simulink model "ThermalRct"  (R2023b)
settings: Solver=FixedStepAuto  StartTime=0.0  StopTime=10.0  RelTol=1e-3
settings Model: DataDictionary=ThermalRct.sldd  Creator=84339  LastModifiedBy=84339
settings OptimizationCC: DefaultParameterBehavior=Inlined  EnhancedBackFolding=on  PassReuseOutputArgsAs=Individual arguments  ZeroExternalMemoryAtStartup=off  ZeroInternalMemoryAtStartup=off  OptimizeBlockOrder=speed  DifferentSizesBufferReuse=on  OptimizationCustomize=off  EfficientTunableParamExpr=on
settings DebuggingCC: ParameterTunabilityLossMsg=error
settings ModelReferenceCC: ModelReferenceNumInstancesAllowed=Single
settings SFSimCC: MATLABDynamicMemAlloc=off
settings RTWCC: Description=Embedded Coder  SystemTargetFile=ert.tlc  EmbeddedCoderDictionary=ASW.sldd  GenCodeOnly=on  TemplateMakefile=ert_default_tmf  DataTypeReplacement=CDataTypesFixedWidth
settings CodeAppCC: ForceParamTrailComments=on  IgnoreCustomStorageClasses=off  OperatorAnnotations=on  SimulinkDataObjDesc=on  SFDataObjDesc=on  InsertBlockDesc=on
settings ERTTargetCC: TargetLangStandard=C99 (ISO)  GenerateSampleERTMain=on  InlinedParameterPlacement=NonHierarchical  ERTCustomFileTemplate=example_file_process.tlc  MaxIdInt64=INT64_MAX  MinIdInt64=INT64_MIN  MaxIdUint64=UINT64_MAX  MaxIdInt32=INT32_MAX  MinIdInt32=INT32_MIN  MaxIdUint32=UINT32_MAX  MaxIdInt16=INT16_MAX  MinIdInt16=INT16_MIN  MaxIdUint16=UINT16_MAX  MaxIdInt8=INT8_MAX  MinIdInt8=INT8_MIN  MaxIdUint8=UINT8_MAX

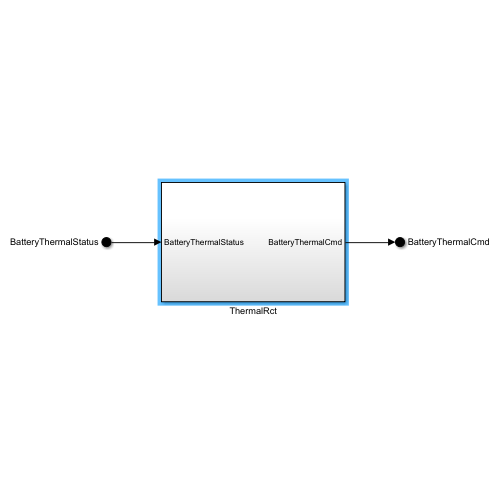
[thumbnail: Simulink's stored preview of the top-level diagram]
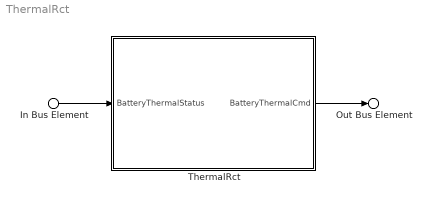
== system ThermalRct ==
  In Bus Element : Inport  PortName=BatteryThermalStatus
  ThermalRct : Subsystem
  Out Bus Element : Outport  PortName=BatteryThermalCmd
  wires:
  ThermalRct/1(BatteryThermalCmd) -> Out Bus Element/1
  In Bus Element/1 -> ThermalRct/1(BatteryThermalStatus)

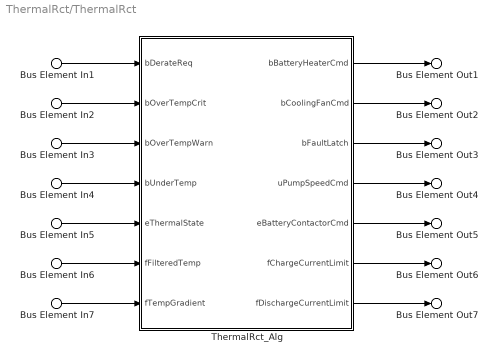
== system ThermalRct/ThermalRct ==
  Bus Element In1 : Inport  PortName=BatteryThermalStatus  Element=bDerateReq
  Bus Element In2 : Inport  PortName=BatteryThermalStatus  Element=bOverTempCrit
  Bus Element In3 : Inport  PortName=BatteryThermalStatus  Element=bOverTempWarn
  Bus Element In4 : Inport  PortName=BatteryThermalStatus  Element=bUnderTemp
  Bus Element In5 : Inport  PortName=BatteryThermalStatus  Element=eThermalState
  Bus Element In6 : Inport  PortName=BatteryThermalStatus  Element=fFilteredTemp
  Bus Element In7 : Inport  PortName=BatteryThermalStatus  Element=fTempGradient
  ThermalRct_Alg : Subsystem
      settings: RTWFcnNameOpts=Use subsystem name
  Bus Element Out2 : Outport  PortName=BatteryThermalCmd  Element=bCoolingFanCmd
  Bus Element Out1 : Outport  PortName=BatteryThermalCmd  Element=bBatteryHeaterCmd
  Bus Element Out3 : Outport  PortName=BatteryThermalCmd  Element=bFaultLatch
  Bus Element Out4 : Outport  PortName=BatteryThermalCmd  Element=uPumpSpeedCmd
  Bus Element Out5 : Outport  PortName=BatteryThermalCmd  Element=eBatteryContactorCmd
  Bus Element Out6 : Outport  PortName=BatteryThermalCmd  Element=fChargeCurrentLimit
  Bus Element Out7 : Outport  PortName=BatteryThermalCmd  Element=fDischargeCurrentLimit
  wires:
  Bus Element In1/1 -> ThermalRct_Alg/1(bDerateReq)
  Bus Element In2/1 -> ThermalRct_Alg/2(bOverTempCrit)
  Bus Element In3/1 -> ThermalRct_Alg/3(bOverTempWarn)
  Bus Element In4/1 -> ThermalRct_Alg/4(bUnderTemp)
  Bus Element In5/1 -> ThermalRct_Alg/5(eThermalState)
  Bus Element In6/1 -> ThermalRct_Alg/6(fFilteredTemp)
  Bus Element In7/1 -> ThermalRct_Alg/7(fTempGradient)
  ThermalRct_Alg/1(bBatteryHeaterCmd) -> Bus Element Out1/1
  ThermalRct_Alg/2(bCoolingFanCmd) -> Bus Element Out2/1
  ThermalRct_Alg/3(bFaultLatch) -> Bus Element Out3/1
  ThermalRct_Alg/4(uPumpSpeedCmd) -> Bus Element Out4/1
  ThermalRct_Alg/5(eBatteryContactorCmd) -> Bus Element Out5/1
  ThermalRct_Alg/6(fChargeCurrentLimit) -> Bus Element Out6/1
  ThermalRct_Alg/7(fDischargeCurrentLimit) -> Bus Element Out7/1

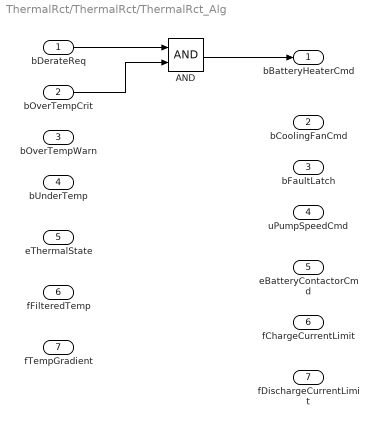
== system ThermalRct/ThermalRct/ThermalRct_Alg ==
  bDerateReq : Inport
  bOverTempCrit : Inport  Port=2
  bOverTempWarn : Inport  Port=3
  bUnderTemp : Inport  Port=4
  eThermalState : Inport  Port=5
  fFilteredTemp : Inport  Port=6
  fTempGradient : Inport  Port=7
  AND : Logic  AllPortsSameDT=off  OutDataTypeStr=boolean
  bBatteryHeaterCmd : Outport
  bCoolingFanCmd : Outport  Port=2
  bFaultLatch : Outport  Port=3
  uPumpSpeedCmd : Outport  Port=4
  eBatteryContactorCmd : Outport  Port=5
  fChargeCurrentLimit : Outport  Port=6
  fDischargeCurrentLimit : Outport  Port=7
  wires:
  bDerateReq/1 -> AND/1
  bOverTempCrit/1 -> AND/2
  AND/1 -> bBatteryHeaterCmd/1
